simulink model "FourWheelSim_base"  (R2021b)
settings: Solver=ode4  StartTime=0.0  StopTime=10  FixedStep=0.001  EnableMultiTasking=on
values from neighbouring files (symbols this model uses):
  a_f = [1.434106444513048,-3.490394354141787e-04,2.761516722659314,6.000050177239062e+04,2.990012596710455e+03,-1.736376596503330e-04,0.526021936511837]    [VehicleParamsFEM20.m]    (also in VehicleParamsFEM20_Gear17.m; VehicleParamsFEM21.m)
  a_r = a_f    [VehicleParamsFEM20.m]    (also in VehicleParamsFEM20_Gear17.m; VehicleParamsFEM21.m)
  afx_f = [1.736519934348130,-2.903281841026900e-04,2.651682004580759,7.000047010028531e+04,3.270011055825476e+03,-0.001252141095807,1.596836353939939]    [VehicleParamsFEM20.m]    (also in VehicleParamsFEM20_Gear17.m; VehicleParamsFEM21.m)
  afx_r = afx_f    [VehicleParamsFEM20.m]    (also in VehicleParamsFEM20_Gear17.m; VehicleParamsFEM21.m)
  agx_f = [0.230000000000000,2.936116597489246e+04,7.137436879966481e+03,0,0]    [VehicleParamsFEM20.m]    (also in VehicleParamsFEM20_Gear17.m; VehicleParamsFEM21.m)
  agx_r = agx_f    [VehicleParamsFEM20.m]    (also in VehicleParamsFEM20_Gear17.m; VehicleParamsFEM21.m)
  agy_f = [0.852564208514954,3.000069064154418e+04,2.070023877794581e+03,-5.089267464508360e-04,0.519364283925805]    [VehicleParamsFEM20.m]    (also in VehicleParamsFEM20_Gear17.m; VehicleParamsFEM21.m)
  agy_r = agy_f    [VehicleParamsFEM20.m]    (also in VehicleParamsFEM20_Gear17.m; VehicleParamsFEM21.m)
  b_f = [3.436650779629654,1.566044221042620e-05,0.028598122547093,3.408741969645286e+03,5.995144285148312e+03,-1.736376595720277e-04,0.526021936449385]    [VehicleParamsFEM20.m]    (also in VehicleParamsFEM20_Gear17.m; VehicleParamsFEM21.m)
  Brake_Factor = 0.66    [VehicleParamsFEM20.m]    (also in VehicleParamsFEM20_Gear17.m; VehicleParamsFEM21.m)
  Cd = Cd/(40/3.6)^2    (= 0.6885)    [VehicleParamsFEM20.m]    (also in VehicleParamsFEM20_Gear17.m; VehicleParamsFEM21.m)
  CLF = DFf/40/40    (= 0.06)    [VehicleParamsFEM20.m]    (also in VehicleParamsFEM20_Gear17.m; VehicleParamsFEM21.m)
  CLR = DFr/40/40    (= 0.065)    [VehicleParamsFEM20.m]    (also in VehicleParamsFEM20_Gear17.m; VehicleParamsFEM21.m)
  cPiston_Area_F = 2*pi*(0.0254/2)^2    (= 0.00101341495819)    [VehicleParamsFEM20.m]    (also in VehicleParamsFEM20_Gear17.m; VehicleParamsFEM21.m)
  cPiston_Area_R = 2*pi*(0.0254/2)^2    (= 0.00101341495819)    [VehicleParamsFEM20.m]    (also in VehicleParamsFEM20_Gear17.m; VehicleParamsFEM21.m)
  delta = 15.5    [VehicleParamsFEM20.m]    (also in VehicleParamsFEM20_Gear17.m; VehicleParamsFEM21.m)
  df = 1.225    [VehicleParamsFEM20.m]    (also in VehicleParamsFEM20_Gear17.m; VehicleParamsFEM21.m)
  dr = 1.225    [VehicleParamsFEM20.m]    (also in VehicleParamsFEM20_Gear17.m; VehicleParamsFEM21.m)
  eff_Radius_F = (180/2-13.5)/1000    (= 0.0765)    [VehicleParamsFEM20.m]    (also in VehicleParamsFEM20_Gear17.m; VehicleParamsFEM21.m)
  eff_Radius_R = (180/2-13.5)/1000    (= 0.0765)    [VehicleParamsFEM20.m]    (also in VehicleParamsFEM20_Gear17.m; VehicleParamsFEM21.m)
  Fd = 60*2    (= 120)    [VehicleParamsFEM20.m]    (also in VehicleParamsFEM20_Gear17.m; VehicleParamsFEM21.m)
  Frtoe = 0    [VehicleParamsFEM20.m]    (also in VehicleParamsFEM20_Gear17.m; VehicleParamsFEM21.m)
  gear_f = 13.75    [VehicleParamsFEM20.m]    (also in VehicleParamsFEM20_Gear17.m = 14.45; VehicleParamsFEM21.m)
  gear_r = 13.75    [VehicleParamsFEM20.m]    (also in VehicleParamsFEM20_Gear17.m = 14.45; VehicleParamsFEM21.m)
  hg = 0.28    [VehicleParamsFEM20.m]    (also in VehicleParamsFEM20_Gear17.m; VehicleParamsFEM21.m)
  HV_voltage = 600    [VehicleParamsFEM20.m]    (also in VehicleParamsFEM20_Gear17.m; VehicleParamsFEM21.m)
  I = 112    [VehicleParamsFEM20.m]    (also in VehicleParamsFEM20_Gear17.m; VehicleParamsFEM21.m)
  ini_v = ini_speed/3.6    (= 10.4166666667)    [VehicleParamsFEM20.m]    (also in VehicleParamsFEM20_Gear17.m; VehicleParamsFEM21.m)
  Kframe = 5.94*10^6    (= 5940000)    [VehicleParamsFEM20.m]    (also in VehicleParamsFEM20_Gear17.m; VehicleParamsFEM21.m)
  kk_f = 2800*180/pi    (= 160428.182637)    [VehicleParamsFEM20.m]    (also in VehicleParamsFEM20_Gear17.m; VehicleParamsFEM21.m)
  kk_r = 4200*180/pi    (= 240642.273955)    [VehicleParamsFEM20.m]    (also in VehicleParamsFEM20_Gear17.m; VehicleParamsFEM21.m)
  krfr = 0.5    [VehicleParamsFEM20.m]    (also in VehicleParamsFEM20_Gear17.m; VehicleParamsFEM21.m)
  l = 1.530    (= 1.53)    [VehicleParamsFEM20.m]    (also in VehicleParamsFEM20_Gear17.m; VehicleParamsFEM21.m)
  lf = l*(1-WBf)    (= 0.7956)    [VehicleParamsFEM20.m]    (also in VehicleParamsFEM20_Gear17.m; VehicleParamsFEM21.m)
  lr = l*WBf    (= 0.7344)    [VehicleParamsFEM20.m]    (also in VehicleParamsFEM20_Gear17.m; VehicleParamsFEM21.m)
  M = 200+60    (= 260)    [VehicleParamsFEM20.m]    (also in VehicleParamsFEM20_Gear17.m; VehicleParamsFEM21.m)
  mu_tire_F = 0.587-0.587+0.55    (= 0.55)    [VehicleParamsFEM20.m]    (also in VehicleParamsFEM20_Gear17.m; VehicleParamsFEM21.m)
  mu_tire_R = 0.587-0.587+0.55    (= 0.55)    [VehicleParamsFEM20.m]    (also in VehicleParamsFEM20_Gear17.m; VehicleParamsFEM21.m)
  Mwf = Iwf/Rwf/Rwf    (= 3.82716814816)    [VehicleParamsFEM20.m]    (also in VehicleParamsFEM20_Gear17.m; VehicleParamsFEM21.m)
  Mwr = Iwr/Rwr/Rwr    (= 3.82716814816)    [VehicleParamsFEM20.m]    (also in VehicleParamsFEM20_Gear17.m; VehicleParamsFEM21.m)
  rcf = 0.000    (= 0)    [VehicleParamsFEM20.m]    (also in VehicleParamsFEM20_Gear17.m; VehicleParamsFEM21.m = 15)
  rch = rcf*WBf+rcr*(1-WBf)    (= 0)    [VehicleParamsFEM20.m]    (also in VehicleParamsFEM20_Gear17.m; VehicleParamsFEM21.m = 22.8)
  rcr = 0.000    (= 0)    [VehicleParamsFEM20.m]    (also in VehicleParamsFEM20_Gear17.m; VehicleParamsFEM21.m = 30)
  Reartoe = -2    [VehicleParamsFEM20.m]    (also in VehicleParamsFEM20_Gear17.m; VehicleParamsFEM21.m)
  Rr_toe = Reartoe*pi/180    (= -0.0349065850399)    [VehicleParamsFEM20.m]    (also in VehicleParamsFEM20_Gear17.m; VehicleParamsFEM21.m)
  Rwf = 18*(25.4/1000)/2    (= 0.2286)    [VehicleParamsFEM20.m]    (also in VehicleParamsFEM20_Gear17.m; VehicleParamsFEM21.m)
  Rwr = 18*(25.4/1000)/2    (= 0.2286)    [VehicleParamsFEM20.m]    (also in VehicleParamsFEM20_Gear17.m; VehicleParamsFEM21.m)
  T_TireF = TireL_f/V    (= 0.036760000032)    [VehicleParamsFEM20.m]    (also in VehicleParamsFEM20_Gear17.m; VehicleParamsFEM21.m)
  T_TireR = TireL_r/V    (= 0.036760000032)    [VehicleParamsFEM20.m]    (also in VehicleParamsFEM20_Gear17.m; VehicleParamsFEM21.m)
  tspeed = 37.5    [VehicleParamsFEM20.m]    (also in VehicleParamsFEM20_Gear17.m; VehicleParamsFEM21.m)
  WBf = 0.48    [VehicleParamsFEM20.m]    (also in VehicleParamsFEM20_Gear17.m; VehicleParamsFEM21.m)
  zc_f = castrail_Fr/1000    (= 0)    [VehicleParamsFEM20.m]    (also in VehicleParamsFEM20_Gear17.m; VehicleParamsFEM21.m)
  zc_r = castrail_Rr/1000    (= 0)    [VehicleParamsFEM20.m]    (also in VehicleParamsFEM20_Gear17.m; VehicleParamsFEM21.m)
libraries: simulink x25, dspstat3 x1
(part 3 of 4)

== system FourWheelSim_base/TractiveSystem/Sensors/differentialGPS ==
  X : Inport
  Add : Sum  Inputs=+-
  Constant6 : Constant  Value=0.001
  Delay19 : Delay  DelayLength=1
  Divide : Product  Inputs=*/
  X' : Outport  VectorParamsAs1DForOutWhenUnconnected=off
  wires:
  Add/1 -> Divide/1
  Constant6/1 -> Divide/2
  Divide/1 -> X'/1
  X/1 -> Delay19/1, Add/1
  Delay19/1 -> Add/2

== system FourWheelSim_base/TractiveSystem/Sensors/differentialGPS1 ==
  X : Inport
  Add : Sum  Inputs=+-
  Constant6 : Constant  Value=0.001
  Delay19 : Delay  DelayLength=1
  Divide : Product  Inputs=*/
  X' : Outport  VectorParamsAs1DForOutWhenUnconnected=off
  wires:
  Delay19/1 -> Add/2
  X/1 -> Add/1, Delay19/1
  Divide/1 -> X'/1
  Constant6/1 -> Divide/2
  Add/1 -> Divide/1

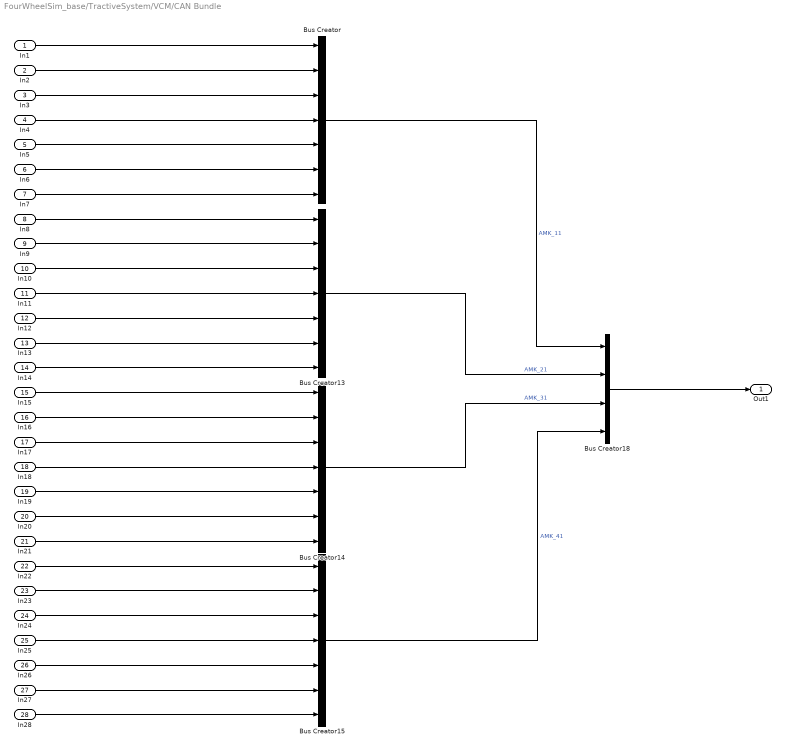
== system FourWheelSim_base/TractiveSystem/VCM/CAN Bundle ==
  In1 : Inport
  In2 : Inport  Port=2
  In3 : Inport  Port=3
  In4 : Inport  Port=4
  In5 : Inport  Port=5
  In6 : Inport  Port=6
  In7 : Inport  Port=7
  In8 : Inport  Port=8
  In9 : Inport  Port=9
  In10 : Inport  Port=10
  In11 : Inport  Port=11
  In12 : Inport  Port=12
  In13 : Inport  Port=13
  In14 : Inport  Port=14
  In15 : Inport  Port=15
  In16 : Inport  Port=16
  In17 : Inport  Port=17
  In18 : Inport  Port=18
  In19 : Inport  Port=19
  In20 : Inport  Port=20
  In21 : Inport  Port=21
  In22 : Inport  Port=22
  In23 : Inport  Port=23
  In24 : Inport  Port=24
  In25 : Inport  Port=25
  In26 : Inport  Port=26
  In27 : Inport  Port=27
  In28 : Inport  Port=28
  Bus Creator{,13..15} (4 alike) : BusCreator  Inputs=7
  Bus Creator18 : BusCreator  Inputs=4
  Out1 : Outport  VectorParamsAs1DForOutWhenUnconnected=off
  wires:
  In7/1 -> Bus Creator/7
  In6/1 -> Bus Creator/6
  In5/1 -> Bus Creator/5
  In4/1 -> Bus Creator/4
  In3/1 -> Bus Creator/3
  In2/1 -> Bus Creator/2
  In1/1 -> Bus Creator/1
  Bus Creator18/1 -> Out1/1
  In8/1 -> Bus Creator13/1
  In18/1 -> Bus Creator14/4
  In13/1 -> Bus Creator13/6
  In28/1 -> Bus Creator15/7
  Bus Creator14/1 -> Bus Creator18/3  "AMK_31"
  In19/1 -> Bus Creator14/5
  In22/1 -> Bus Creator15/1
  In11/1 -> Bus Creator13/4
  Bus Creator/1 -> Bus Creator18/1  "AMK_11"
  In26/1 -> Bus Creator15/5
  In27/1 -> Bus Creator15/6
  In23/1 -> Bus Creator15/2
  In14/1 -> Bus Creator13/7
  In21/1 -> Bus Creator14/7
  Bus Creator15/1 -> Bus Creator18/4  "AMK_41"
  In17/1 -> Bus Creator14/3
  In25/1 -> Bus Creator15/4
  Bus Creator13/1 -> Bus Creator18/2  "AMK_21"
  In20/1 -> Bus Creator14/6
  In15/1 -> Bus Creator14/1
  In9/1 -> Bus Creator13/2
  In10/1 -> Bus Creator13/3
  In24/1 -> Bus Creator15/3
  In16/1 -> Bus Creator14/2
  In12/1 -> Bus Creator13/5

== system FourWheelSim_base/TractiveSystem/VCM/speedlimit ==
  rpm : Inport
  kph : Inport  Port=2
  Min : MinMax  Inputs=2
  kph to motor rpm : Subsystem
  speedlimit(rpm) : Outport  VectorParamsAs1DForOutWhenUnconnected=off
  wires:
  kph to motor rpm/1(rpm) -> Min/2
  rpm/1 -> Min/1
  Min/1 -> speedlimit(rpm)/1
  kph/1 -> kph to motor rpm/1(kph)

== system FourWheelSim_base/4-wheel Vehicle model/comb slip model/Load/RL Load Diff ==
  note: VD講座第9回参照
  note: 横加速度による荷重移動
  FrontLoad : Inport
  RearLoad : Inport  Port=2
  LatG : Inport  Port=3
  Front Load Diff : Gain  Gain=M/df*(krfr*(hg-rch)+(1-WBf)*rcf)
  Gain : Gain  Gain=-1
  Gain1 : Gain  Gain=-1
  Rear_Load Diff1 : Gain  Gain=M/dr*((1-krfr)*(hg-rch)+WBf*rcr)
  Saturation Dynamic : simulink/Discontinuities/Saturation Dynamic  OutMin=[]  OutMax=[]  OutDataTypeStr=Inherit: Same as second input  OutDataType=fixdt(1, 16)  OutScaling=2^-10  DoSatur=off
  Saturation Dynamic2 : simulink/Discontinuities/Saturation Dynamic  OutMin=[]  OutMax=[]  OutDataTypeStr=Inherit: Same as second input  OutDataType=fixdt(1, 16)  OutScaling=2^-10  DoSatur=off
  Front Load Diff_RL : Outport  VectorParamsAs1DForOutWhenUnconnected=off
  Rear Load Diff_RL : Outport  Port=2  VectorParamsAs1DForOutWhenUnconnected=off
  wires:
  Gain1/1 -> Saturation Dynamic2/3
  Saturation Dynamic/1 -> Front Load Diff_RL/1
  LatG/1 -> Front Load Diff/1, Rear_Load Diff1/1
  RearLoad/1 -> Saturation Dynamic2/1, Gain1/1
  Rear_Load Diff1/1 -> Saturation Dynamic2/2
  FrontLoad/1 -> Gain/1, Saturation Dynamic/1
  Gain/1 -> Saturation Dynamic/3
  Front Load Diff/1 -> Saturation Dynamic/2
  Saturation Dynamic2/1 -> Rear Load Diff_RL/1

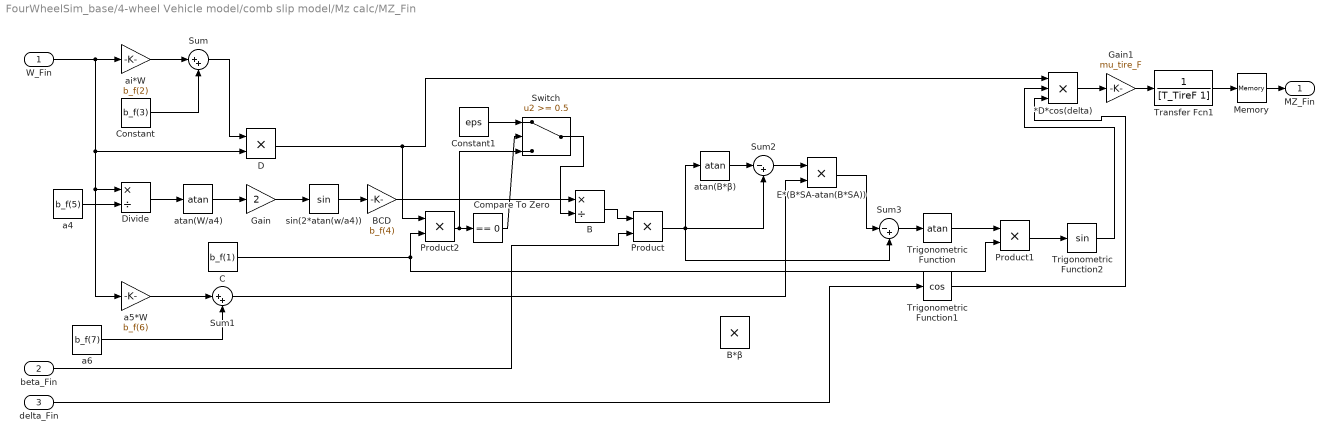
== system FourWheelSim_base/4-wheel Vehicle model/comb slip model/Mz calc/MZ_Fin ==
  W_Fin : Inport
  beta_Fin : Inport  Port=2
  delta_Fin : Inport  Port=3
  *D*cos(delta) : Product  Inputs=3  RndMeth=Zero
  B : Product  Inputs=*/
  B*β : Product  Inputs=**
  BCD : Gain  Gain=b_f(4)
  C : Constant  Value=b_f(1)
  Compare To Zero : simulink/Logic and Bit Operations/Compare To Zero  relop===  OutDataTypeStr=boolean
  Constant : Constant  Value=b_f(3)
  Constant1 : Constant  Value=eps
  D : Product  RndMeth=Zero
  Divide : Product  Inputs=*/
  E*(B*SA-atan(B*SA)) : Product  RndMeth=Zero
  Gain : Gain  Gain=2
  Gain1 : Gain  Gain=mu_tire_F
  Memory : Memory
  Product : Product  RndMeth=Zero
  Product1 : Product  RndMeth=Zero
  Product2 : Product
  Sum : Sum  Inputs=|++
  Sum1 : Sum  Inputs=|++
  Sum2 : Sum  Inputs=|-+
  Sum3 : Sum  Inputs=|-+
  Switch : Switch  Threshold=0.5
  Transfer Fcn1 : TransferFcn  Denominator=[T_TireF 1]
  Trigonometric Function : Trigonometry  Operator=atan
  Trigonometric Function1 : Trigonometry  Operator=cos
  Trigonometric Function2 : Trigonometry
  a4 : Constant  Value=b_f(5)
  a5*W : Gain  Gain=b_f(6)
  a6 : Constant  Value=b_f(7)
  ai*W : Gain  Gain=b_f(2)
  atan(B*β) : Trigonometry  Operator=atan
  atan(W/a4) : Trigonometry  Operator=atan
  sin(2*atan(w/a4)) : Trigonometry
  MZ_Fin : Outport  VectorParamsAs1DForOutWhenUnconnected=off
  wires:
  Constant/1 -> Sum/2
  ai*W/1 -> Sum/1
  Sum/1 -> D/1
  a4/1 -> Divide/2
  Divide/1 -> atan(W/a4)/1
  atan(W/a4)/1 -> Gain/1
  Gain/1 -> sin(2*atan(w/a4))/1
  sin(2*atan(w/a4))/1 -> BCD/1
  BCD/1 -> B/1
  C/1 -> Product1/2, Product2/2
  a5*W/1 -> Sum1/1
  a6/1 -> Sum1/2
  B/1 -> Product/1
  beta_Fin/1 -> Product/2
  Sum1/1 -> E*(B*SA-atan(B*SA))/2
  Sum3/1 -> Trigonometric Function/1
  D/1 -> Product2/1, *D*cos(delta)/1
  Gain1/1 -> Transfer Fcn1/1
  delta_Fin/1 -> Trigonometric Function1/1
  Trigonometric Function1/1 -> *D*cos(delta)/3
  Trigonometric Function/1 -> Product1/1
  Trigonometric Function2/1 -> *D*cos(delta)/2
  Product1/1 -> Trigonometric Function2/1
  W_Fin/1 -> a5*W/1, Divide/1, D/2, ai*W/1
  Product2/1 -> Switch/3, Compare To Zero/1
  Compare To Zero/1 -> Switch/2
  Constant1/1 -> Switch/1
  Switch/1 -> B/2
  *D*cos(delta)/1 -> Gain1/1
  Transfer Fcn1/1 -> Memory/1
  Memory/1 -> MZ_Fin/1
  Product/1 -> Sum2/2, Sum3/2, atan(B*β)/1
  atan(B*β)/1 -> Sum2/1
  Sum2/1 -> E*(B*SA-atan(B*SA))/1
  E*(B*SA-atan(B*SA))/1 -> Sum3/1

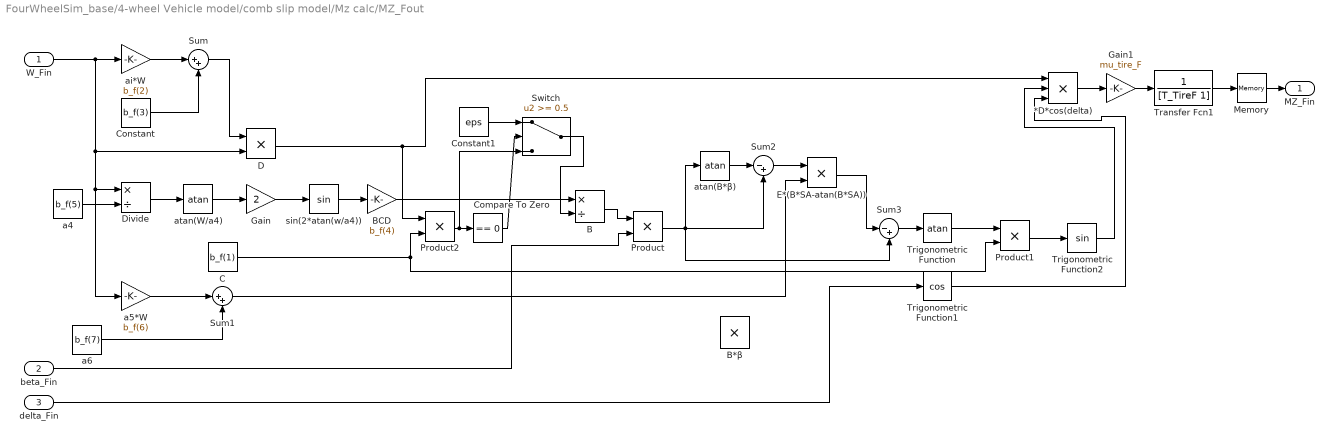
== system FourWheelSim_base/4-wheel Vehicle model/comb slip model/Mz calc/MZ_Fout ==
  W_Fin : Inport
  beta_Fin : Inport  Port=2
  delta_Fin : Inport  Port=3
  *D*cos(delta) : Product  Inputs=3  RndMeth=Zero
  B : Product  Inputs=*/
  B*β : Product  Inputs=**
  BCD : Gain  Gain=b_f(4)
  C : Constant  Value=b_f(1)
  Compare To Zero : simulink/Logic and Bit Operations/Compare To Zero  relop===  OutDataTypeStr=boolean
  Constant : Constant  Value=b_f(3)
  Constant1 : Constant  Value=eps
  D : Product  RndMeth=Zero
  Divide : Product  Inputs=*/
  E*(B*SA-atan(B*SA)) : Product  RndMeth=Zero
  Gain : Gain  Gain=2
  Gain1 : Gain  Gain=mu_tire_F
  Memory : Memory
  Product : Product  RndMeth=Zero
  Product1 : Product  RndMeth=Zero
  Product2 : Product
  Sum : Sum  Inputs=|++
  Sum1 : Sum  Inputs=|++
  Sum2 : Sum  Inputs=|-+
  Sum3 : Sum  Inputs=|-+
  Switch : Switch  Threshold=0.5
  Transfer Fcn1 : TransferFcn  Denominator=[T_TireF 1]
  Trigonometric Function : Trigonometry  Operator=atan
  Trigonometric Function1 : Trigonometry  Operator=cos
  Trigonometric Function2 : Trigonometry
  a4 : Constant  Value=b_f(5)
  a5*W : Gain  Gain=b_f(6)
  a6 : Constant  Value=b_f(7)
  ai*W : Gain  Gain=b_f(2)
  atan(B*β) : Trigonometry  Operator=atan
  atan(W/a4) : Trigonometry  Operator=atan
  sin(2*atan(w/a4)) : Trigonometry
  MZ_Fin : Outport  VectorParamsAs1DForOutWhenUnconnected=off
  wires:
  Constant/1 -> Sum/2
  ai*W/1 -> Sum/1
  Sum/1 -> D/1
  a4/1 -> Divide/2
  Divide/1 -> atan(W/a4)/1
  atan(W/a4)/1 -> Gain/1
  Gain/1 -> sin(2*atan(w/a4))/1
  sin(2*atan(w/a4))/1 -> BCD/1
  BCD/1 -> B/1
  C/1 -> Product1/2, Product2/2
  a5*W/1 -> Sum1/1
  a6/1 -> Sum1/2
  B/1 -> Product/1
  beta_Fin/1 -> Product/2
  Sum1/1 -> E*(B*SA-atan(B*SA))/2
  Sum3/1 -> Trigonometric Function/1
  D/1 -> Product2/1, *D*cos(delta)/1
  Gain1/1 -> Transfer Fcn1/1
  delta_Fin/1 -> Trigonometric Function1/1
  Trigonometric Function1/1 -> *D*cos(delta)/3
  Trigonometric Function/1 -> Product1/1
  Trigonometric Function2/1 -> *D*cos(delta)/2
  Product1/1 -> Trigonometric Function2/1
  W_Fin/1 -> a5*W/1, Divide/1, D/2, ai*W/1
  Product2/1 -> Switch/3, Compare To Zero/1
  Compare To Zero/1 -> Switch/2
  Constant1/1 -> Switch/1
  Switch/1 -> B/2
  *D*cos(delta)/1 -> Gain1/1
  Transfer Fcn1/1 -> Memory/1
  Memory/1 -> MZ_Fin/1
  Product/1 -> Sum2/2, Sum3/2, atan(B*β)/1
  atan(B*β)/1 -> Sum2/1
  Sum2/1 -> E*(B*SA-atan(B*SA))/1
  E*(B*SA-atan(B*SA))/1 -> Sum3/1

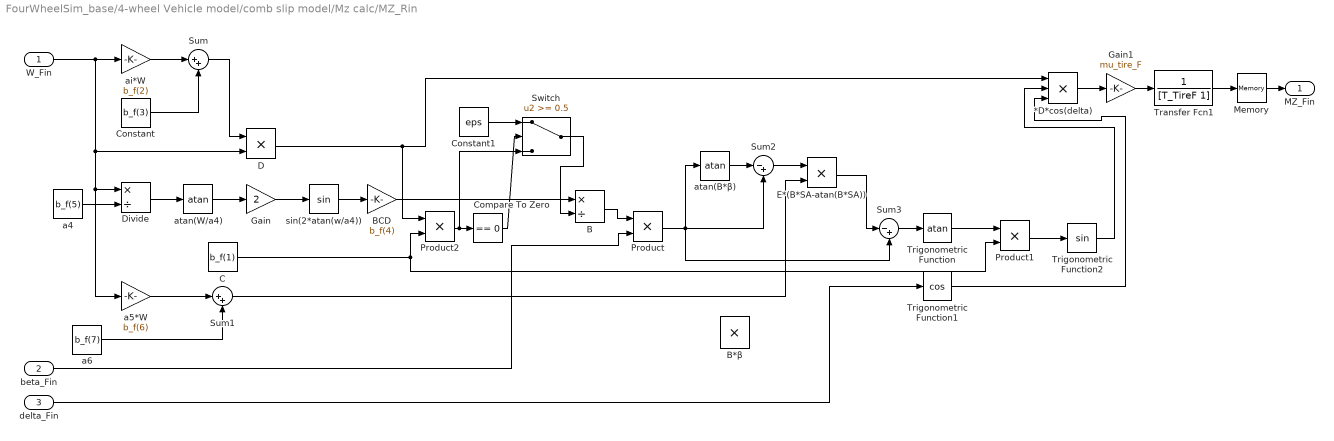
== system FourWheelSim_base/4-wheel Vehicle model/comb slip model/Mz calc/MZ_Rin ==
  W_Fin : Inport
  beta_Fin : Inport  Port=2
  delta_Fin : Inport  Port=3
  *D*cos(delta) : Product  Inputs=3  RndMeth=Zero
  B : Product  Inputs=*/
  B*β : Product  Inputs=**
  BCD : Gain  Gain=b_f(4)
  C : Constant  Value=b_f(1)
  Compare To Zero : simulink/Logic and Bit Operations/Compare To Zero  relop===  OutDataTypeStr=boolean
  Constant : Constant  Value=b_f(3)
  Constant1 : Constant  Value=eps
  D : Product  RndMeth=Zero
  Divide : Product  Inputs=*/
  E*(B*SA-atan(B*SA)) : Product  RndMeth=Zero
  Gain : Gain  Gain=2
  Gain1 : Gain  Gain=mu_tire_F
  Memory : Memory
  Product : Product  RndMeth=Zero
  Product1 : Product  RndMeth=Zero
  Product2 : Product
  Sum : Sum  Inputs=|++
  Sum1 : Sum  Inputs=|++
  Sum2 : Sum  Inputs=|-+
  Sum3 : Sum  Inputs=|-+
  Switch : Switch  Threshold=0.5
  Transfer Fcn1 : TransferFcn  Denominator=[T_TireF 1]
  Trigonometric Function : Trigonometry  Operator=atan
  Trigonometric Function1 : Trigonometry  Operator=cos
  Trigonometric Function2 : Trigonometry
  a4 : Constant  Value=b_f(5)
  a5*W : Gain  Gain=b_f(6)
  a6 : Constant  Value=b_f(7)
  ai*W : Gain  Gain=b_f(2)
  atan(B*β) : Trigonometry  Operator=atan
  atan(W/a4) : Trigonometry  Operator=atan
  sin(2*atan(w/a4)) : Trigonometry
  MZ_Fin : Outport  VectorParamsAs1DForOutWhenUnconnected=off
  wires:
  Constant/1 -> Sum/2
  ai*W/1 -> Sum/1
  Sum/1 -> D/1
  a4/1 -> Divide/2
  Divide/1 -> atan(W/a4)/1
  atan(W/a4)/1 -> Gain/1
  Gain/1 -> sin(2*atan(w/a4))/1
  sin(2*atan(w/a4))/1 -> BCD/1
  BCD/1 -> B/1
  C/1 -> Product1/2, Product2/2
  a5*W/1 -> Sum1/1
  a6/1 -> Sum1/2
  B/1 -> Product/1
  beta_Fin/1 -> Product/2
  Sum1/1 -> E*(B*SA-atan(B*SA))/2
  Sum3/1 -> Trigonometric Function/1
  D/1 -> Product2/1, *D*cos(delta)/1
  Gain1/1 -> Transfer Fcn1/1
  delta_Fin/1 -> Trigonometric Function1/1
  Trigonometric Function1/1 -> *D*cos(delta)/3
  Trigonometric Function/1 -> Product1/1
  Trigonometric Function2/1 -> *D*cos(delta)/2
  Product1/1 -> Trigonometric Function2/1
  W_Fin/1 -> a5*W/1, Divide/1, D/2, ai*W/1
  Product2/1 -> Switch/3, Compare To Zero/1
  Compare To Zero/1 -> Switch/2
  Constant1/1 -> Switch/1
  Switch/1 -> B/2
  *D*cos(delta)/1 -> Gain1/1
  Transfer Fcn1/1 -> Memory/1
  Memory/1 -> MZ_Fin/1
  Product/1 -> Sum2/2, Sum3/2, atan(B*β)/1
  atan(B*β)/1 -> Sum2/1
  Sum2/1 -> E*(B*SA-atan(B*SA))/1
  E*(B*SA-atan(B*SA))/1 -> Sum3/1

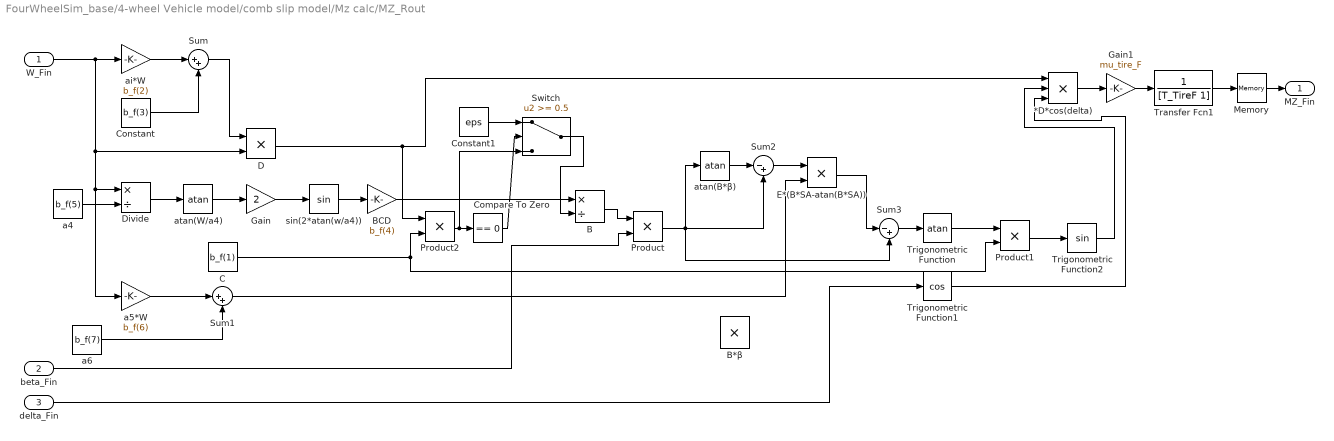
== system FourWheelSim_base/4-wheel Vehicle model/comb slip model/Mz calc/MZ_Rout ==
  W_Fin : Inport
  beta_Fin : Inport  Port=2
  delta_Fin : Inport  Port=3
  *D*cos(delta) : Product  Inputs=3  RndMeth=Zero
  B : Product  Inputs=*/
  B*β : Product  Inputs=**
  BCD : Gain  Gain=b_f(4)
  C : Constant  Value=b_f(1)
  Compare To Zero : simulink/Logic and Bit Operations/Compare To Zero  relop===  OutDataTypeStr=boolean
  Constant : Constant  Value=b_f(3)
  Constant1 : Constant  Value=eps
  D : Product  RndMeth=Zero
  Divide : Product  Inputs=*/
  E*(B*SA-atan(B*SA)) : Product  RndMeth=Zero
  Gain : Gain  Gain=2
  Gain1 : Gain  Gain=mu_tire_F
  Memory : Memory
  Product : Product  RndMeth=Zero
  Product1 : Product  RndMeth=Zero
  Product2 : Product
  Sum : Sum  Inputs=|++
  Sum1 : Sum  Inputs=|++
  Sum2 : Sum  Inputs=|-+
  Sum3 : Sum  Inputs=|-+
  Switch : Switch  Threshold=0.5
  Transfer Fcn1 : TransferFcn  Denominator=[T_TireF 1]
  Trigonometric Function : Trigonometry  Operator=atan
  Trigonometric Function1 : Trigonometry  Operator=cos
  Trigonometric Function2 : Trigonometry
  a4 : Constant  Value=b_f(5)
  a5*W : Gain  Gain=b_f(6)
  a6 : Constant  Value=b_f(7)
  ai*W : Gain  Gain=b_f(2)
  atan(B*β) : Trigonometry  Operator=atan
  atan(W/a4) : Trigonometry  Operator=atan
  sin(2*atan(w/a4)) : Trigonometry
  MZ_Fin : Outport  VectorParamsAs1DForOutWhenUnconnected=off
  wires:
  Constant/1 -> Sum/2
  ai*W/1 -> Sum/1
  Sum/1 -> D/1
  a4/1 -> Divide/2
  Divide/1 -> atan(W/a4)/1
  atan(W/a4)/1 -> Gain/1
  Gain/1 -> sin(2*atan(w/a4))/1
  sin(2*atan(w/a4))/1 -> BCD/1
  BCD/1 -> B/1
  C/1 -> Product1/2, Product2/2
  a5*W/1 -> Sum1/1
  a6/1 -> Sum1/2
  B/1 -> Product/1
  beta_Fin/1 -> Product/2
  Sum1/1 -> E*(B*SA-atan(B*SA))/2
  Sum3/1 -> Trigonometric Function/1
  D/1 -> Product2/1, *D*cos(delta)/1
  Gain1/1 -> Transfer Fcn1/1
  delta_Fin/1 -> Trigonometric Function1/1
  Trigonometric Function1/1 -> *D*cos(delta)/3
  Trigonometric Function/1 -> Product1/1
  Trigonometric Function2/1 -> *D*cos(delta)/2
  Product1/1 -> Trigonometric Function2/1
  W_Fin/1 -> a5*W/1, Divide/1, D/2, ai*W/1
  Product2/1 -> Switch/3, Compare To Zero/1
  Compare To Zero/1 -> Switch/2
  Constant1/1 -> Switch/1
  Switch/1 -> B/2
  *D*cos(delta)/1 -> Gain1/1
  Transfer Fcn1/1 -> Memory/1
  Memory/1 -> MZ_Fin/1
  Product/1 -> Sum2/2, Sum3/2, atan(B*β)/1
  atan(B*β)/1 -> Sum2/1
  Sum2/1 -> E*(B*SA-atan(B*SA))/1
  E*(B*SA-atan(B*SA))/1 -> Sum3/1

== system FourWheelSim_base/4-wheel Vehicle model/comb slip model/comb Fx calc/Force_Fin_comb_FX ==
  W_Fin : Inport
  beta_Fin : Inport  Port=2
  slip rate : Inport  Port=3
  *D : Product  RndMeth=Zero
  B : Product  Inputs=*/
  BCD : Gain  Gain=agx_f(2)
  C : Constant  Value=agx_f(1)
  Compare To Zero : simulink/Logic and Bit Operations/Compare To Zero  relop===  OutDataTypeStr=boolean
  Constant1 : Constant  Value=eps
  Divide : Product  Inputs=*/
  E*(B*SA-atan(B*SA)) : Product  RndMeth=Zero
  Gain : Gain  Gain=2
  Gain1 : Gain  Gain=mu_tire_F
  Product : Product  RndMeth=Zero
  Product1 : Product  RndMeth=Zero
  Product2 : Product
  Scope : Scope
  Sum1 : Sum  Inputs=|++
  Sum2 : Sum  Inputs=|-+
  Sum3 : Sum  Inputs=|-+
  Switch : Switch  Threshold=0.5
  Tire Force : Subsystem
  Trigonometric Function : Trigonometry  Operator=atan
  Trigonometric Function2 : Trigonometry  Operator=cos
  a4 : Constant  Value=agx_f(3)
  a5*W : Gain  Gain=agy_f(4)
  a6 : Constant  Value=agx_f(5)
  atan(B*β) : Trigonometry  Operator=atan
  atan(W/a4) : Trigonometry  Operator=atan
  sin(2*atan(w/a4)) : Trigonometry
  Force_Fin : Outport  VectorParamsAs1DForOutWhenUnconnected=off
  wires:
  a4/1 -> Divide/2
  Divide/1 -> atan(W/a4)/1
  atan(W/a4)/1 -> Gain/1
  Gain/1 -> sin(2*atan(w/a4))/1
  sin(2*atan(w/a4))/1 -> BCD/1
  C/1 -> Product1/2, Product2/2
  a5*W/1 -> Sum1/1
  a6/1 -> Sum1/2
  B/1 -> Product/1
  Sum1/1 -> E*(B*SA-atan(B*SA))/2
  Sum3/1 -> Trigonometric Function/1
  Trigonometric Function/1 -> Product1/1
  Trigonometric Function2/1 -> *D/2
  Product1/1 -> Trigonometric Function2/1
  W_Fin/1 -> Tire Force/1(Load), Scope/1, a5*W/1, Divide/1
  *D/1 -> Gain1/1
  Gain1/1 -> Force_Fin/1
  Product/1 -> Sum2/2, Sum3/2, atan(B*β)/1
  atan(B*β)/1 -> Sum2/1
  Sum2/1 -> E*(B*SA-atan(B*SA))/1
  E*(B*SA-atan(B*SA))/1 -> Sum3/1
  Tire Force/1(Force_Rear) -> Product2/1, *D/1
  Product2/1 -> Switch/3, Compare To Zero/1
  Constant1/1 -> Switch/1
  Switch/1 -> B/2
  Compare To Zero/1 -> Switch/2
  BCD/1 -> B/1
  slip rate/1 -> Tire Force/2(Slip Rate)
  beta_Fin/1 -> Product/2

== system FourWheelSim_base/4-wheel Vehicle model/comb slip model/comb Fx calc/Force_Fout_comb_FX ==
  W_Fout : Inport
  beta_Fout : Inport  Port=2
  slip rate : Inport  Port=3
  *D : Product  RndMeth=Zero
  B : Product  Inputs=*/
  BCD : Gain  Gain=agx_f(2)
  C : Constant  Value=agx_f(1)
  Compare To Zero : simulink/Logic and Bit Operations/Compare To Zero  relop===  OutDataTypeStr=boolean
  Constant1 : Constant  Value=eps
  Divide : Product  Inputs=*/
  E*(B*SA-atan(B*SA)) : Product  RndMeth=Zero
  Gain : Gain  Gain=2
  Gain1 : Gain  Gain=mu_tire_F
  Product : Product  RndMeth=Zero
  Product1 : Product  RndMeth=Zero
  Product2 : Product
  Sum1 : Sum  Inputs=|++
  Sum2 : Sum  Inputs=|-+
  Sum3 : Sum  Inputs=|-+
  Switch : Switch  Threshold=0.5
  Tire Force : Subsystem
  Trigonometric Function : Trigonometry  Operator=atan
  Trigonometric Function2 : Trigonometry  Operator=cos
  a4 : Constant  Value=agx_f(3)
  a5*W : Gain  Gain=agy_f(4)
  a6 : Constant  Value=agx_f(5)
  atan(B*β) : Trigonometry  Operator=atan
  atan(W/a4) : Trigonometry  Operator=atan
  sin(2*atan(w/a4)) : Trigonometry
  Force_Fout : Outport  VectorParamsAs1DForOutWhenUnconnected=off
  wires:
  a4/1 -> Divide/2
  Divide/1 -> atan(W/a4)/1
  atan(W/a4)/1 -> Gain/1
  Gain/1 -> sin(2*atan(w/a4))/1
  sin(2*atan(w/a4))/1 -> BCD/1
  C/1 -> Product1/2, Product2/2
  a5*W/1 -> Sum1/1
  a6/1 -> Sum1/2
  B/1 -> Product/1
  Sum1/1 -> E*(B*SA-atan(B*SA))/2
  Sum3/1 -> Trigonometric Function/1
  Trigonometric Function/1 -> Product1/1
  Trigonometric Function2/1 -> *D/2
  Product1/1 -> Trigonometric Function2/1
  W_Fout/1 -> Tire Force/1(Load), a5*W/1, Divide/1
  *D/1 -> Gain1/1
  Product/1 -> Sum2/2, Sum3/2, atan(B*β)/1
  atan(B*β)/1 -> Sum2/1
  Sum2/1 -> E*(B*SA-atan(B*SA))/1
  E*(B*SA-atan(B*SA))/1 -> Sum3/1
  Tire Force/1(Force_Rear) -> Product2/1, *D/1
  Product2/1 -> Switch/3, Compare To Zero/1
  Constant1/1 -> Switch/1
  Switch/1 -> B/2
  Compare To Zero/1 -> Switch/2
  BCD/1 -> B/1
  slip rate/1 -> Tire Force/2(Slip Rate)
  beta_Fout/1 -> Product/2
  Gain1/1 -> Force_Fout/1

== system FourWheelSim_base/4-wheel Vehicle model/comb slip model/comb Fx calc/Force_Rin_comb_FX ==
  W_Rin : Inport
  beta_Rin : Inport  Port=2
  slip rate : Inport  Port=3
  *D : Product  RndMeth=Zero
  B : Product  Inputs=*/
  BCD : Gain  Gain=agx_r(2)
  C : Constant  Value=agx_r(1)
  Compare To Zero : simulink/Logic and Bit Operations/Compare To Zero  relop===  OutDataTypeStr=boolean
  Constant1 : Constant  Value=eps
  Divide : Product  Inputs=*/
  E*(B*SA-atan(B*SA)) : Product  RndMeth=Zero
  Gain : Gain  Gain=2
  Gain1 : Gain  Gain=mu_tire_R
  Product : Product  RndMeth=Zero
  Product1 : Product  RndMeth=Zero
  Product2 : Product
  Sum1 : Sum  Inputs=|++
  Sum2 : Sum  Inputs=|-+
  Sum3 : Sum  Inputs=|-+
  Switch : Switch  Threshold=0.5
  Tire Force : Subsystem
  Trigonometric Function : Trigonometry  Operator=atan
  Trigonometric Function2 : Trigonometry  Operator=cos
  a4 : Constant  Value=agx_r(3)
  a5*W : Gain  Gain=agy_r(4)
  a6 : Constant  Value=agx_r(5)
  atan(B*β) : Trigonometry  Operator=atan
  atan(W/a4) : Trigonometry  Operator=atan
  sin(2*atan(w/a4)) : Trigonometry
  Force_Rin : Outport  VectorParamsAs1DForOutWhenUnconnected=off
  wires:
  a4/1 -> Divide/2
  Divide/1 -> atan(W/a4)/1
  atan(W/a4)/1 -> Gain/1
  Gain/1 -> sin(2*atan(w/a4))/1
  sin(2*atan(w/a4))/1 -> BCD/1
  C/1 -> Product1/2, Product2/2
  a5*W/1 -> Sum1/1
  a6/1 -> Sum1/2
  B/1 -> Product/1
  Sum1/1 -> E*(B*SA-atan(B*SA))/2
  Sum3/1 -> Trigonometric Function/1
  Trigonometric Function/1 -> Product1/1
  Trigonometric Function2/1 -> *D/2
  Product1/1 -> Trigonometric Function2/1
  W_Rin/1 -> Tire Force/1(Load), a5*W/1, Divide/1
  Product/1 -> Sum2/2, Sum3/2, atan(B*β)/1
  atan(B*β)/1 -> Sum2/1
  Sum2/1 -> E*(B*SA-atan(B*SA))/1
  E*(B*SA-atan(B*SA))/1 -> Sum3/1
  Tire Force/1(Force_Rear) -> Product2/1, *D/1
  Product2/1 -> Switch/3, Compare To Zero/1
  Constant1/1 -> Switch/1
  Switch/1 -> B/2
  Compare To Zero/1 -> Switch/2
  BCD/1 -> B/1
  slip rate/1 -> Tire Force/2(Slip Rate)
  beta_Rin/1 -> Product/2
  Gain1/1 -> Force_Rin/1
  *D/1 -> Gain1/1

== system FourWheelSim_base/4-wheel Vehicle model/comb slip model/comb Fx calc/Force_Rout_comb1_FX ==
  W_Rout : Inport
  beta_Rout : Inport  Port=2
  slip rate : Inport  Port=3
  *D : Product  RndMeth=Zero
  B : Product  Inputs=*/
  BCD : Gain  Gain=agx_r(2)
  C : Constant  Value=agx_r(1)
  Compare To Zero : simulink/Logic and Bit Operations/Compare To Zero  relop===  OutDataTypeStr=boolean
  Constant1 : Constant  Value=eps
  Divide : Product  Inputs=*/
  E*(B*SA-atan(B*SA)) : Product  RndMeth=Zero
  Gain : Gain  Gain=2
  Gain1 : Gain  Gain=mu_tire_R
  Product : Product  RndMeth=Zero
  Product1 : Product  RndMeth=Zero
  Product2 : Product
  Scope : Scope
  Sum1 : Sum  Inputs=|++
  Sum2 : Sum  Inputs=|-+
  Sum3 : Sum  Inputs=|-+
  Switch : Switch  Threshold=0.5
  Tire Force : Subsystem
  Trigonometric Function : Trigonometry  Operator=atan
  Trigonometric Function2 : Trigonometry  Operator=cos
  a4 : Constant  Value=agx_r(3)
  a5*W : Gain  Gain=agy_r(4)
  a6 : Constant  Value=agx_r(5)
  atan(B*β) : Trigonometry  Operator=atan
  atan(W/a4) : Trigonometry  Operator=atan
  sin(2*atan(w/a4)) : Trigonometry
  Force_Rin : Outport  VectorParamsAs1DForOutWhenUnconnected=off
  wires:
  a4/1 -> Divide/2
  Divide/1 -> Scope/1, atan(W/a4)/1
  atan(W/a4)/1 -> Gain/1
  Gain/1 -> sin(2*atan(w/a4))/1
  sin(2*atan(w/a4))/1 -> BCD/1
  C/1 -> Product1/2, Product2/2
  a5*W/1 -> Sum1/1
  a6/1 -> Sum1/2
  B/1 -> Product/1
  Sum1/1 -> E*(B*SA-atan(B*SA))/2
  Sum3/1 -> Trigonometric Function/1
  Trigonometric Function/1 -> Product1/1
  Trigonometric Function2/1 -> *D/2
  Product1/1 -> Trigonometric Function2/1
  W_Rout/1 -> Tire Force/1(Load), a5*W/1, Divide/1
  Product/1 -> Sum2/2, Sum3/2, atan(B*β)/1
  atan(B*β)/1 -> Sum2/1
  Sum2/1 -> E*(B*SA-atan(B*SA))/1
  E*(B*SA-atan(B*SA))/1 -> Sum3/1
  Tire Force/1(Force_Rear) -> Product2/1, *D/1
  Product2/1 -> Switch/3, Compare To Zero/1
  Constant1/1 -> Switch/1
  Switch/1 -> B/2
  Compare To Zero/1 -> Switch/2
  BCD/1 -> B/1
  slip rate/1 -> Tire Force/2(Slip Rate)
  beta_Rout/1 -> Product/2
  Gain1/1 -> Force_Rin/1
  *D/1 -> Gain1/1

== system FourWheelSim_base/4-wheel Vehicle model/comb slip model/comb Fy calc/Force_Fin_comb_FY ==
  note: C = agy_f(1);
      | D = PureY;
      | E = Load*agy_f(4) + agy_f(5);
      | B = agy_f(2)*sin(2*atan(Load/agy_f(3)))/(D*C);
      | Fy = D*cos(C*atan(B*SlipAngle-E*(B*SlipAngle-atan(B*SlipAngle))));
  W_Fin : Inport
  beta_Fin : Inport  Port=2
  slip rate : Inport  Port=3
  *D : Product  RndMeth=Zero
  B : Product  Inputs=*/
  BCD : Gain  Gain=agy_f(2)
  C : Constant  Value=agy_f(1)
  Compare To Zero : simulink/Logic and Bit Operations/Compare To Zero  relop===  OutDataTypeStr=boolean
  Constant1 : Constant  Value=eps
  Divide : Product  Inputs=*/
  E*(B*SA-atan(B*SA)) : Product  RndMeth=Zero
  Force_Fin_Pure : Subsystem
  Gain : Gain  Gain=2
  Gain1 : Gain  Gain=-mu_tire_F
  Product : Product  RndMeth=Zero
  Product1 : Product  RndMeth=Zero
  Product2 : Product
  Sum1 : Sum  Inputs=|++
  Sum2 : Sum  Inputs=|-+
  Sum3 : Sum  Inputs=|-+
  Switch : Switch  Threshold=0.5
  Transfer Fcn1 : TransferFcn  Denominator=[T_TireF 1]
  Trigonometric Function : Trigonometry  Operator=atan
  Trigonometric Function2 : Trigonometry  Operator=cos
  a4 : Constant  Value=agy_f(3)
  a5*W : Gain  Gain=agy_f(4)
  a6 : Constant  Value=agy_f(5)
  atan(B*β) : Trigonometry  Operator=atan
  atan(W/a4) : Trigonometry  Operator=atan
  sin(2*atan(w/a4)) : Trigonometry
  Force_Fin : Outport  VectorParamsAs1DForOutWhenUnconnected=off
  wires:
  a4/1 -> Divide/2
  Divide/1 -> atan(W/a4)/1
  atan(W/a4)/1 -> Gain/1
  Gain/1 -> sin(2*atan(w/a4))/1
  sin(2*atan(w/a4))/1 -> BCD/1
  C/1 -> Product1/2, Product2/2
  a5*W/1 -> Sum1/1
  a6/1 -> Sum1/2
  B/1 -> Product/1
  beta_Fin/1 -> Force_Fin_Pure/2(beta_Fin)
  Sum1/1 -> E*(B*SA-atan(B*SA))/2
  Sum3/1 -> Trigonometric Function/1
  Gain1/1 -> Transfer Fcn1/1
  Trigonometric Function/1 -> Product1/1
  Trigonometric Function2/1 -> *D/2
  Product1/1 -> Trigonometric Function2/1
  W_Fin/1 -> Force_Fin_Pure/1(W_Fin), a5*W/1, Divide/1
  *D/1 -> Gain1/1
  Transfer Fcn1/1 -> Force_Fin/1
  Product/1 -> Sum2/2, Sum3/2, atan(B*β)/1
  atan(B*β)/1 -> Sum2/1
  Sum2/1 -> E*(B*SA-atan(B*SA))/1
  E*(B*SA-atan(B*SA))/1 -> Sum3/1
  Force_Fin_Pure/1(Force_Fin_Pure) -> Product2/1, *D/1
  slip rate/1 -> Product/2
  Product2/1 -> Switch/3, Compare To Zero/1
  Constant1/1 -> Switch/1
  Switch/1 -> B/2
  Compare To Zero/1 -> Switch/2
  BCD/1 -> B/1

== system FourWheelSim_base/4-wheel Vehicle model/comb slip model/comb Fy calc/Force_Fout_comb_FY ==
  W_Fin : Inport
  beta_Fin : Inport  Port=2
  slip rate : Inport  Port=3
  *D : Product  RndMeth=Zero
  B : Product  Inputs=*/
  BCD : Gain  Gain=agy_f(2)
  C : Constant  Value=agy_f(1)
  Compare To Zero : simulink/Logic and Bit Operations/Compare To Zero  relop===  OutDataTypeStr=boolean
  Constant1 : Constant  Value=eps
  Divide : Product  Inputs=*/
  E*(B*SA-atan(B*SA)) : Product  RndMeth=Zero
  Force_Fout_Pure : Subsystem
  Gain : Gain  Gain=2
  Gain1 : Gain  Gain=-mu_tire_F
  Product : Product  RndMeth=Zero
  Product1 : Product  RndMeth=Zero
  Product2 : Product
  Sum1 : Sum  Inputs=|++
  Sum2 : Sum  Inputs=|-+
  Sum3 : Sum  Inputs=|-+
  Switch : Switch  Threshold=0.5
  Transfer Fcn1 : TransferFcn  Denominator=[T_TireF 1]
  Trigonometric Function : Trigonometry  Operator=atan
  Trigonometric Function2 : Trigonometry  Operator=cos
  a4 : Constant  Value=agy_f(3)
  a5*W : Gain  Gain=agy_f(4)
  a6 : Constant  Value=agy_f(5)
  atan(B*β) : Trigonometry  Operator=atan
  atan(W/a4) : Trigonometry  Operator=atan
  sin(2*atan(w/a4)) : Trigonometry
  Force_Fout : Outport  VectorParamsAs1DForOutWhenUnconnected=off
  wires:
  a4/1 -> Divide/2
  Divide/1 -> atan(W/a4)/1
  atan(W/a4)/1 -> Gain/1
  Gain/1 -> sin(2*atan(w/a4))/1
  sin(2*atan(w/a4))/1 -> BCD/1
  C/1 -> Product1/2, Product2/2
  a5*W/1 -> Sum1/1
  a6/1 -> Sum1/2
  B/1 -> Product/1
  beta_Fin/1 -> Force_Fout_Pure/2(beta_Fin)
  Sum1/1 -> E*(B*SA-atan(B*SA))/2
  Sum3/1 -> Trigonometric Function/1
  Gain1/1 -> Transfer Fcn1/1
  Trigonometric Function/1 -> Product1/1
  Trigonometric Function2/1 -> *D/2
  Product1/1 -> Trigonometric Function2/1
  W_Fin/1 -> Force_Fout_Pure/1(W_Fin), a5*W/1, Divide/1
  *D/1 -> Gain1/1
  Transfer Fcn1/1 -> Force_Fout/1
  Product/1 -> Sum2/2, Sum3/2, atan(B*β)/1
  atan(B*β)/1 -> Sum2/1
  Sum2/1 -> E*(B*SA-atan(B*SA))/1
  E*(B*SA-atan(B*SA))/1 -> Sum3/1
  Force_Fout_Pure/1(Force_Fout_Pure) -> Product2/1, *D/1
  slip rate/1 -> Product/2
  Product2/1 -> Switch/3, Compare To Zero/1
  Constant1/1 -> Switch/1
  Switch/1 -> B/2
  Compare To Zero/1 -> Switch/2
  BCD/1 -> B/1

== system FourWheelSim_base/4-wheel Vehicle model/comb slip model/comb Fy calc/Force_Rin_comb_FY ==
  W_Fin : Inport
  beta_Fin : Inport  Port=2
  slip rate : Inport  Port=3
  *D : Product  RndMeth=Zero
  B : Product  Inputs=*/
  BCD : Gain  Gain=agy_r(2)
  C : Constant  Value=agy_r(1)
  Compare To Zero : simulink/Logic and Bit Operations/Compare To Zero  relop===  OutDataTypeStr=boolean
  Constant1 : Constant  Value=eps
  Divide : Product  Inputs=*/
  E*(B*SA-atan(B*SA)) : Product  RndMeth=Zero
  "Force_Rin_Pure " : Subsystem
  Gain : Gain  Gain=2
  Gain1 : Gain  Gain=-mu_tire_R
  Product : Product  RndMeth=Zero
  Product1 : Product  RndMeth=Zero
  Product2 : Product
  Sum1 : Sum  Inputs=|++
  Sum2 : Sum  Inputs=|-+
  Sum3 : Sum  Inputs=|-+
  Switch : Switch  Threshold=0.5
  Transfer Fcn1 : TransferFcn  Denominator=[T_TireR 1]
  Trigonometric Function : Trigonometry  Operator=atan
  Trigonometric Function2 : Trigonometry  Operator=cos
  a4 : Constant  Value=agy_r(3)
  a5*W : Gain  Gain=agy_r(4)
  a6 : Constant  Value=agy_r(5)
  atan(B*β) : Trigonometry  Operator=atan
  atan(W/a4) : Trigonometry  Operator=atan
  sin(2*atan(w/a4)) : Trigonometry
  Force_Rin : Outport  VectorParamsAs1DForOutWhenUnconnected=off
  wires:
  a4/1 -> Divide/2
  Divide/1 -> atan(W/a4)/1
  atan(W/a4)/1 -> Gain/1
  Gain/1 -> sin(2*atan(w/a4))/1
  sin(2*atan(w/a4))/1 -> BCD/1
  C/1 -> Product1/2, Product2/2
  a5*W/1 -> Sum1/1
  a6/1 -> Sum1/2
  B/1 -> Product/1
  beta_Fin/1 -> "Force_Rin_Pure "/2(beta_Fin)
  Sum1/1 -> E*(B*SA-atan(B*SA))/2
  Sum3/1 -> Trigonometric Function/1
  Gain1/1 -> Transfer Fcn1/1
  Trigonometric Function/1 -> Product1/1
  Trigonometric Function2/1 -> *D/2
  Product1/1 -> Trigonometric Function2/1
  W_Fin/1 -> "Force_Rin_Pure "/1(W_Fin), a5*W/1, Divide/1
  *D/1 -> Gain1/1
  Transfer Fcn1/1 -> Force_Rin/1
  Product/1 -> Sum2/2, Sum3/2, atan(B*β)/1
  atan(B*β)/1 -> Sum2/1
  Sum2/1 -> E*(B*SA-atan(B*SA))/1
  E*(B*SA-atan(B*SA))/1 -> Sum3/1
  "Force_Rin_Pure "/1(Force_Rin_Pure) -> Product2/1, *D/1
  slip rate/1 -> Product/2
  Product2/1 -> Switch/3, Compare To Zero/1
  Constant1/1 -> Switch/1
  Switch/1 -> B/2
  Compare To Zero/1 -> Switch/2
  BCD/1 -> B/1

== system FourWheelSim_base/4-wheel Vehicle model/comb slip model/comb Fy calc/Force_Rout_comb_FY ==
  W_Fin : Inport
  beta_Fin : Inport  Port=2
  slip rate : Inport  Port=3
  *D : Product  RndMeth=Zero
  B : Product  Inputs=*/
  BCD : Gain  Gain=agy_r(2)
  C : Constant  Value=agy_r(1)
  Compare To Zero : simulink/Logic and Bit Operations/Compare To Zero  relop===  OutDataTypeStr=boolean
  Constant1 : Constant  Value=eps
  Divide : Product  Inputs=*/
  E*(B*SA-atan(B*SA)) : Product  RndMeth=Zero
  "Force_Rout_Pure " : Subsystem
  Gain : Gain  Gain=2
  Gain1 : Gain  Gain=-mu_tire_R
  Product : Product  RndMeth=Zero
  Product1 : Product  RndMeth=Zero
  Product2 : Product
  Sum1 : Sum  Inputs=|++
  Sum2 : Sum  Inputs=|-+
  Sum3 : Sum  Inputs=|-+
  Switch : Switch  Threshold=0.5
  Transfer Fcn1 : TransferFcn  Denominator=[T_TireR 1]
  Trigonometric Function : Trigonometry  Operator=atan
  Trigonometric Function2 : Trigonometry  Operator=cos
  a4 : Constant  Value=agy_r(3)
  a5*W : Gain  Gain=agy_r(4)
  a6 : Constant  Value=agy_r(5)
  atan(B*β) : Trigonometry  Operator=atan
  atan(W/a4) : Trigonometry  Operator=atan
  sin(2*atan(w/a4)) : Trigonometry
  Force_Rout : Outport  VectorParamsAs1DForOutWhenUnconnected=off
  wires:
  a4/1 -> Divide/2
  Divide/1 -> atan(W/a4)/1
  atan(W/a4)/1 -> Gain/1
  Gain/1 -> sin(2*atan(w/a4))/1
  sin(2*atan(w/a4))/1 -> BCD/1
  C/1 -> Product1/2, Product2/2
  a5*W/1 -> Sum1/1
  a6/1 -> Sum1/2
  B/1 -> Product/1
  beta_Fin/1 -> "Force_Rout_Pure "/2(beta_Fin)
  Sum1/1 -> E*(B*SA-atan(B*SA))/2
  Sum3/1 -> Trigonometric Function/1
  Gain1/1 -> Transfer Fcn1/1
  Trigonometric Function/1 -> Product1/1
  Trigonometric Function2/1 -> *D/2
  Product1/1 -> Trigonometric Function2/1
  W_Fin/1 -> "Force_Rout_Pure "/1(W_Fin), a5*W/1, Divide/1
  *D/1 -> Gain1/1
  Transfer Fcn1/1 -> Force_Rout/1
  Product/1 -> Sum2/2, Sum3/2, atan(B*β)/1
  atan(B*β)/1 -> Sum2/1
  Sum2/1 -> E*(B*SA-atan(B*SA))/1
  E*(B*SA-atan(B*SA))/1 -> Sum3/1
  "Force_Rout_Pure "/1(Force_Rout_Pure) -> Product2/1, *D/1
  slip rate/1 -> Product/2
  Product2/1 -> Switch/3, Compare To Zero/1
  Constant1/1 -> Switch/1
  Switch/1 -> B/2
  Compare To Zero/1 -> Switch/2
  BCD/1 -> B/1

== system FourWheelSim_base/TractiveSystem/VCM/speedlimit/kph to motor rpm ==
  kph : Inport
  Gear : Gain  Gain=13.75
  to m/s : Gain  Gain=1000/3600
  toTire_rpm : Gain  Gain=60/(2*pi*0.228)
  rpm : Outport  VectorParamsAs1DForOutWhenUnconnected=off
  wires:
  Gear/1 -> rpm/1
  to m/s/1 -> toTire_rpm/1
  toTire_rpm/1 -> Gear/1
  kph/1 -> to m/s/1

== system FourWheelSim_base/4-wheel Vehicle model/comb slip model/comb Fx calc/Force_Fin_comb_FX/Tire Force ==
  Load : Inport
  Slip Rate : Inport  Port=2
  *D*cos(delta) : Product  RndMeth=Zero
  B : Product  Inputs=*/
  BCD : Gain  Gain=afx_f(4)
  C : Constant  Value=afx_f(1)
  Compare To Zero : simulink/Logic and Bit Operations/Compare To Zero  relop===  OutDataTypeStr=boolean
  Constant : Constant  Value=afx_f(3)
  Constant1 : Constant  Value=eps
  D : Product  RndMeth=Zero
  Divide : Product  Inputs=*/
  E*(B*SA-atan(B*SA)) : Product  RndMeth=Zero
  Gain : Gain  Gain=2
  Product : Product  RndMeth=Zero
  Product1 : Product  RndMeth=Zero
  Product2 : Product
  Sum : Sum  Inputs=|++
  Sum1 : Sum  Inputs=|++
  Sum2 : Sum  Inputs=|-+
  Sum3 : Sum  Inputs=|-+
  Switch : Switch  Threshold=0.5
  Trigonometric Function : Trigonometry  Operator=atan
  Trigonometric Function2 : Trigonometry
  a4 : Constant  Value=afx_f(5)
  a5*W : Gain  Gain=afx_f(6)
  a6 : Constant  Value=afx_f(7)
  ai*W : Gain  Gain=afx_f(2)
  atan(B*β) : Trigonometry  Operator=atan
  atan(W/a4) : Trigonometry  Operator=atan
  sin(2*atan(w/a4)) : Trigonometry
  Force_Rear : Outport  VectorParamsAs1DForOutWhenUnconnected=off
  wires:
  Constant/1 -> Sum/2
  ai*W/1 -> Sum/1
  Sum/1 -> D/1
  a4/1 -> Divide/2
  Divide/1 -> atan(W/a4)/1
  atan(W/a4)/1 -> Gain/1
  Gain/1 -> sin(2*atan(w/a4))/1
  sin(2*atan(w/a4))/1 -> BCD/1
  BCD/1 -> B/1
  C/1 -> Product1/2, Product2/2
  a5*W/1 -> Sum1/1
  a6/1 -> Sum1/2
  B/1 -> Product/1
  Slip Rate/1 -> Product/2
  Sum1/1 -> E*(B*SA-atan(B*SA))/2
  Sum3/1 -> Trigonometric Function/1
  D/1 -> Product2/1, *D*cos(delta)/1
  Trigonometric Function/1 -> Product1/1
  Trigonometric Function2/1 -> *D*cos(delta)/2
  Product1/1 -> Trigonometric Function2/1
  Load/1 -> a5*W/1, Divide/1, D/2, ai*W/1
  Product2/1 -> Switch/3, Compare To Zero/1
  Compare To Zero/1 -> Switch/2
  Constant1/1 -> Switch/1
  Switch/1 -> B/2
  *D*cos(delta)/1 -> Force_Rear/1
  Product/1 -> Sum2/2, Sum3/2, atan(B*β)/1
  atan(B*β)/1 -> Sum2/1
  Sum2/1 -> E*(B*SA-atan(B*SA))/1
  E*(B*SA-atan(B*SA))/1 -> Sum3/1

== system FourWheelSim_base/4-wheel Vehicle model/comb slip model/comb Fx calc/Force_Fout_comb_FX/Tire Force ==
  Load : Inport
  Slip Rate : Inport  Port=2
  *D*cos(delta) : Product  RndMeth=Zero
  B : Product  Inputs=*/
  BCD : Gain  Gain=afx_f(4)
  C : Constant  Value=afx_f(1)
  Compare To Zero : simulink/Logic and Bit Operations/Compare To Zero  relop===  OutDataTypeStr=boolean
  Constant : Constant  Value=afx_f(3)
  Constant1 : Constant  Value=eps
  D : Product  RndMeth=Zero
  Divide : Product  Inputs=*/
  E*(B*SA-atan(B*SA)) : Product  RndMeth=Zero
  Gain : Gain  Gain=2
  Product : Product  RndMeth=Zero
  Product1 : Product  RndMeth=Zero
  Product2 : Product
  Sum : Sum  Inputs=|++
  Sum1 : Sum  Inputs=|++
  Sum2 : Sum  Inputs=|-+
  Sum3 : Sum  Inputs=|-+
  Switch : Switch  Threshold=0.5
  Trigonometric Function : Trigonometry  Operator=atan
  Trigonometric Function2 : Trigonometry
  a4 : Constant  Value=afx_f(5)
  a5*W : Gain  Gain=afx_f(6)
  a6 : Constant  Value=afx_f(7)
  ai*W : Gain  Gain=afx_f(2)
  atan(B*β) : Trigonometry  Operator=atan
  atan(W/a4) : Trigonometry  Operator=atan
  sin(2*atan(w/a4)) : Trigonometry
  Force_Rear : Outport  VectorParamsAs1DForOutWhenUnconnected=off
  wires:
  Constant/1 -> Sum/2
  ai*W/1 -> Sum/1
  Sum/1 -> D/1
  a4/1 -> Divide/2
  Divide/1 -> atan(W/a4)/1
  atan(W/a4)/1 -> Gain/1
  Gain/1 -> sin(2*atan(w/a4))/1
  sin(2*atan(w/a4))/1 -> BCD/1
  BCD/1 -> B/1
  C/1 -> Product1/2, Product2/2
  a5*W/1 -> Sum1/1
  a6/1 -> Sum1/2
  B/1 -> Product/1
  Slip Rate/1 -> Product/2
  Sum1/1 -> E*(B*SA-atan(B*SA))/2
  Sum3/1 -> Trigonometric Function/1
  D/1 -> Product2/1, *D*cos(delta)/1
  Trigonometric Function/1 -> Product1/1
  Trigonometric Function2/1 -> *D*cos(delta)/2
  Product1/1 -> Trigonometric Function2/1
  Load/1 -> a5*W/1, Divide/1, D/2, ai*W/1
  Product2/1 -> Switch/3, Compare To Zero/1
  Compare To Zero/1 -> Switch/2
  Constant1/1 -> Switch/1
  Switch/1 -> B/2
  *D*cos(delta)/1 -> Force_Rear/1
  Product/1 -> Sum2/2, Sum3/2, atan(B*β)/1
  atan(B*β)/1 -> Sum2/1
  Sum2/1 -> E*(B*SA-atan(B*SA))/1
  E*(B*SA-atan(B*SA))/1 -> Sum3/1

== system FourWheelSim_base/4-wheel Vehicle model/comb slip model/comb Fx calc/Force_Rin_comb_FX/Tire Force ==
  Load : Inport
  Slip Rate : Inport  Port=2
  *D*cos(delta) : Product  RndMeth=Zero
  B : Product  Inputs=*/
  BCD : Gain  Gain=afx_r(4)
  C : Constant  Value=afx_r(1)
  Compare To Zero : simulink/Logic and Bit Operations/Compare To Zero  relop===  OutDataTypeStr=boolean
  Constant : Constant  Value=afx_r(3)
  Constant1 : Constant  Value=eps
  D : Product  RndMeth=Zero
  Divide : Product  Inputs=*/
  E*(B*SA-atan(B*SA)) : Product  RndMeth=Zero
  Gain : Gain  Gain=2
  Product : Product  RndMeth=Zero
  Product1 : Product  RndMeth=Zero
  Product2 : Product
  Sum : Sum  Inputs=|++
  Sum1 : Sum  Inputs=|++
  Sum2 : Sum  Inputs=|-+
  Sum3 : Sum  Inputs=|-+
  Switch : Switch  Threshold=0.5
  Trigonometric Function : Trigonometry  Operator=atan
  Trigonometric Function2 : Trigonometry
  a4 : Constant  Value=afx_r(5)
  a5*W : Gain  Gain=afx_r(6)
  a6 : Constant  Value=afx_r(7)
  ai*W : Gain  Gain=afx_r(2)
  atan(B*β) : Trigonometry  Operator=atan
  atan(W/a4) : Trigonometry  Operator=atan
  sin(2*atan(w/a4)) : Trigonometry
  Force_Rear : Outport  VectorParamsAs1DForOutWhenUnconnected=off
  wires:
  Constant/1 -> Sum/2
  ai*W/1 -> Sum/1
  Sum/1 -> D/1
  a4/1 -> Divide/2
  Divide/1 -> atan(W/a4)/1
  atan(W/a4)/1 -> Gain/1
  Gain/1 -> sin(2*atan(w/a4))/1
  sin(2*atan(w/a4))/1 -> BCD/1
  BCD/1 -> B/1
  C/1 -> Product1/2, Product2/2
  a5*W/1 -> Sum1/1
  a6/1 -> Sum1/2
  B/1 -> Product/1
  Slip Rate/1 -> Product/2
  Sum1/1 -> E*(B*SA-atan(B*SA))/2
  Sum3/1 -> Trigonometric Function/1
  D/1 -> Product2/1, *D*cos(delta)/1
  Trigonometric Function/1 -> Product1/1
  Trigonometric Function2/1 -> *D*cos(delta)/2
  Product1/1 -> Trigonometric Function2/1
  Load/1 -> a5*W/1, Divide/1, D/2, ai*W/1
  Product2/1 -> Switch/3, Compare To Zero/1
  Compare To Zero/1 -> Switch/2
  Constant1/1 -> Switch/1
  Switch/1 -> B/2
  *D*cos(delta)/1 -> Force_Rear/1
  Product/1 -> Sum2/2, Sum3/2, atan(B*β)/1
  atan(B*β)/1 -> Sum2/1
  Sum2/1 -> E*(B*SA-atan(B*SA))/1
  E*(B*SA-atan(B*SA))/1 -> Sum3/1

== system FourWheelSim_base/4-wheel Vehicle model/comb slip model/comb Fx calc/Force_Rout_comb1_FX/Tire Force ==
  Load : Inport
  Slip Rate : Inport  Port=2
  *D*cos(delta) : Product  RndMeth=Zero
  B : Product  Inputs=*/
  BCD : Gain  Gain=afx_r(4)
  C : Constant  Value=afx_r(1)
  Compare To Zero : simulink/Logic and Bit Operations/Compare To Zero  relop===  OutDataTypeStr=boolean
  Constant : Constant  Value=afx_r(3)
  Constant1 : Constant  Value=eps
  D : Product  RndMeth=Zero
  Divide : Product  Inputs=*/
  E*(B*SA-atan(B*SA)) : Product  RndMeth=Zero
  Gain : Gain  Gain=2
  Product : Product  RndMeth=Zero
  Product1 : Product  RndMeth=Zero
  Product2 : Product
  Sum : Sum  Inputs=|++
  Sum1 : Sum  Inputs=|++
  Sum2 : Sum  Inputs=|-+
  Sum3 : Sum  Inputs=|-+
  Switch : Switch  Threshold=0.5
  Trigonometric Function : Trigonometry  Operator=atan
  Trigonometric Function2 : Trigonometry
  a4 : Constant  Value=afx_r(5)
  a5*W : Gain  Gain=afx_r(6)
  a6 : Constant  Value=afx_r(7)
  ai*W : Gain  Gain=afx_r(2)
  atan(B*β) : Trigonometry  Operator=atan
  atan(W/a4) : Trigonometry  Operator=atan
  sin(2*atan(w/a4)) : Trigonometry
  Force_Rear : Outport  VectorParamsAs1DForOutWhenUnconnected=off
  wires:
  Constant/1 -> Sum/2
  ai*W/1 -> Sum/1
  Sum/1 -> D/1
  a4/1 -> Divide/2
  Divide/1 -> atan(W/a4)/1
  atan(W/a4)/1 -> Gain/1
  Gain/1 -> sin(2*atan(w/a4))/1
  sin(2*atan(w/a4))/1 -> BCD/1
  BCD/1 -> B/1
  C/1 -> Product1/2, Product2/2
  a5*W/1 -> Sum1/1
  a6/1 -> Sum1/2
  B/1 -> Product/1
  Slip Rate/1 -> Product/2
  Sum1/1 -> E*(B*SA-atan(B*SA))/2
  Sum3/1 -> Trigonometric Function/1
  D/1 -> Product2/1, *D*cos(delta)/1
  Trigonometric Function/1 -> Product1/1
  Trigonometric Function2/1 -> *D*cos(delta)/2
  Product1/1 -> Trigonometric Function2/1
  Load/1 -> a5*W/1, Divide/1, D/2, ai*W/1
  Product2/1 -> Switch/3, Compare To Zero/1
  Compare To Zero/1 -> Switch/2
  Constant1/1 -> Switch/1
  Switch/1 -> B/2
  *D*cos(delta)/1 -> Force_Rear/1
  Product/1 -> Sum2/2, Sum3/2, atan(B*β)/1
  atan(B*β)/1 -> Sum2/1
  Sum2/1 -> E*(B*SA-atan(B*SA))/1
  E*(B*SA-atan(B*SA))/1 -> Sum3/1

== system FourWheelSim_base/4-wheel Vehicle model/comb slip model/comb Fy calc/Force_Fin_comb_FY/Force_Fin_Pure ==
  note: C = a_f(1);
      | D = (Load*a_f(2) + a_f(3))*Load;
      | E = Load*a_f(6) + a_f(7);
      | B = a_f(4)*sin(2*atan(Load/a_f(5)))/(D*C);
      | PureFy = D*sin(C*atan(B*SlipRate-E*(B*SlipRate-atan(B*SlipRate))));
  W_Fin : Inport
  beta_Fin : Inport  Port=2
  *D*cos(delta) : Product  RndMeth=Zero
  B : Product  Inputs=*/
  B*β : Product  Inputs=**
  BCD : Gain  Gain=a_f(4)
  C : Constant  Value=a_f(1)
  Compare To Zero : simulink/Logic and Bit Operations/Compare To Zero  relop===  OutDataTypeStr=boolean
  Constant : Constant  Value=a_f(3)
  Constant1 : Constant  Value=eps
  D : Product  RndMeth=Zero
  Divide : Product  Inputs=*/
  E*(B*SA-atan(B*SA)) : Product  RndMeth=Zero
  Gain : Gain  Gain=2
  Product : Product  RndMeth=Zero
  Product1 : Product  RndMeth=Zero
  Product2 : Product
  Sum : Sum  Inputs=|++
  Sum1 : Sum  Inputs=|++
  Sum2 : Sum  Inputs=|-+
  Sum3 : Sum  Inputs=|-+
  Switch : Switch  Threshold=0.5
  Trigonometric Function : Trigonometry  Operator=atan
  Trigonometric Function2 : Trigonometry
  a4 : Constant  Value=a_f(5)
  a5*W : Gain  Gain=a_f(6)
  a6 : Constant  Value=a_f(7)
  ai*W : Gain  Gain=a_f(2)
  atan(B*β) : Trigonometry  Operator=atan
  atan(W/a4) : Trigonometry  Operator=atan
  sin(2*atan(w/a4)) : Trigonometry
  Force_Fin_Pure : Outport  VectorParamsAs1DForOutWhenUnconnected=off
  wires:
  Constant/1 -> Sum/2
  ai*W/1 -> Sum/1
  Sum/1 -> D/1
  a4/1 -> Divide/2
  Divide/1 -> atan(W/a4)/1
  atan(W/a4)/1 -> Gain/1
  Gain/1 -> sin(2*atan(w/a4))/1
  sin(2*atan(w/a4))/1 -> BCD/1
  BCD/1 -> B/1
  C/1 -> Product1/2, Product2/2
  a5*W/1 -> Sum1/1
  a6/1 -> Sum1/2
  B/1 -> Product/1
  beta_Fin/1 -> Product/2
  Sum1/1 -> E*(B*SA-atan(B*SA))/2
  Sum3/1 -> Trigonometric Function/1
  D/1 -> Product2/1, *D*cos(delta)/1  "D"
  Trigonometric Function/1 -> Product1/1
  Trigonometric Function2/1 -> *D*cos(delta)/2
  Product1/1 -> Trigonometric Function2/1
  W_Fin/1 -> a5*W/1, Divide/1, D/2, ai*W/1
  Product2/1 -> Switch/3, Compare To Zero/1
  Compare To Zero/1 -> Switch/2
  Constant1/1 -> Switch/1
  Switch/1 -> B/2
  *D*cos(delta)/1 -> Force_Fin_Pure/1
  Product/1 -> Sum2/2, Sum3/2, atan(B*β)/1
  atan(B*β)/1 -> Sum2/1
  Sum2/1 -> E*(B*SA-atan(B*SA))/1
  E*(B*SA-atan(B*SA))/1 -> Sum3/1
